simulink model "post_data_run"  (R2020a)
settings: Solver=FixedStepDiscrete  StartTime=0.0  StopTime=P.t_end  FixedStep=P.dt  RelTol=1e-3  EnableMultiTasking=on
PostLoadFcn:
  | load_post_DC
StopFcn:
  | post_post_DC
settings Model: ExtModeTrigDuration=10000  Creator=divad  LastModifiedBy=divad
settings SolverCC: PositivePriorityOrder=on
settings DataIOCC: ReturnWorkspaceOutputs=off
settings OptimizationCC: LifeSpan=inf
settings DebuggingCC: ArithmeticOperatorsInVariantConditions=warning
settings SFSimCC: SimUseLocalCustomCode=off  CustomCodeUndefinedFunction=UseInterfaceOnly
settings RTWCC: Description=QUARC Win64 Target  SystemTargetFile=quarc_win64.tlc  TemplateMakefile=quarc_default_tmf  RTWUseLocalCustomCode=off
settings CodeAppCC: StateflowObjectComments=on
settings STFCustomTargetCC: TargetPreCompLibLocation=C:\PROGRA~3\QUARC\lib\2020a\win64\release  TargetLangStandard=C99 (ISO)  ConcurrentExecutionCompliant=on  GRTInterface=on  SystemTargetFile=quarc_win64.tlc
settings GRTTargetCC: TargetPreCompLibLocation=C:\PROGRA~3\QUARC\lib\2020a\win64\release  ParMdlRefBuildCompliant=off  CompOptLevelCompliant=off  CombineOutputUpdateFcns=off  MatFileLogging=off  CPPClassGenCompliant=off  GRTInterface=on  UseToolchainInfoCompliant=off  ExtMode=on  ExtModeMexFile=quarc_comm
settings ConfigComp: CovMetricSettings=dswe

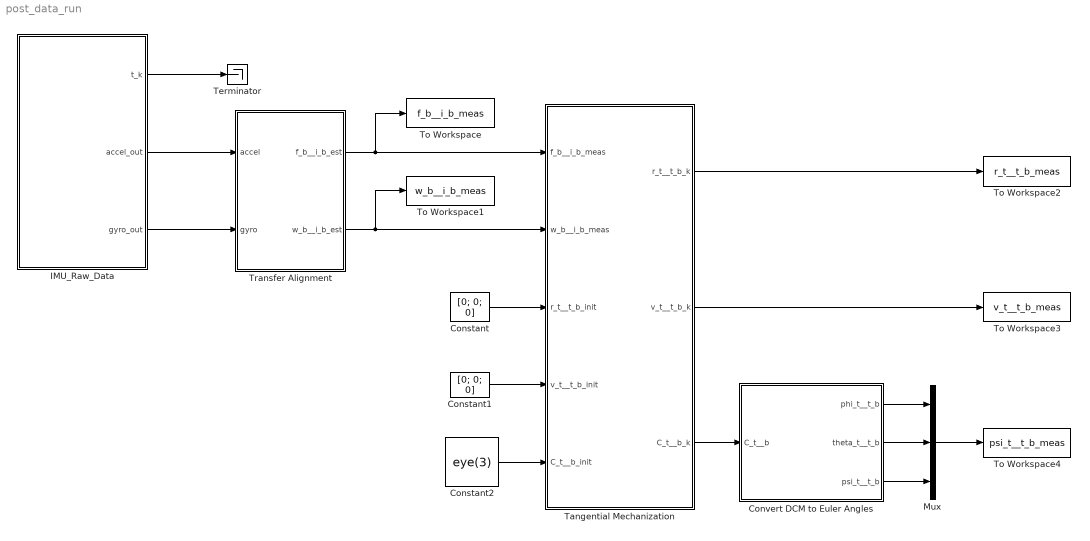
== system post_data_run ==
  Constant : Constant  Value=[0; 0; 0]
  Constant1 : Constant  Value=[0; 0; 0]
  Constant2 : Constant  Value=eye(3)
  Convert DCM to Euler Angles : MATLAB Function  TreatAsAtomicUnit=on
  IMU_Raw_Data : MATLAB Function  TreatAsAtomicUnit=on
  Mux : Mux  Inputs=3
  Tangential Mechanization : Subsystem
  Terminator : Terminator
  To Workspace : ToWorkspace  VariableName=f_b__i_b_meas  SampleTime=-1
      settings: Save2DSignal=2-D array (concatenate along first dimension)
  To Workspace1 : ToWorkspace  VariableName=w_b__i_b_meas  SampleTime=-1
      settings: Save2DSignal=2-D array (concatenate along first dimension)
  To Workspace2 : ToWorkspace  VariableName=r_t__t_b_meas  SampleTime=-1
      settings: Save2DSignal=2-D array (concatenate along first dimension)
  To Workspace3 : ToWorkspace  VariableName=v_t__t_b_meas  SampleTime=-1
      settings: Save2DSignal=2-D array (concatenate along first dimension)
  To Workspace4 : ToWorkspace  VariableName=psi_t__t_b_meas  SampleTime=-1
      settings: Save2DSignal=2-D array (concatenate along first dimension)
  Transfer Alignment : MATLAB Function  TreatAsAtomicUnit=on
  wires:
  IMU_Raw_Data/2(accel_out) -> Transfer Alignment/1(accel)
  IMU_Raw_Data/3(gyro_out) -> Transfer Alignment/2(gyro)
  Transfer Alignment/1(f_b__i_b_est) -> Tangential Mechanization/1(f_b__i_b_meas), To Workspace/1
  Transfer Alignment/2(w_b__i_b_est) -> To Workspace1/1, Tangential Mechanization/2(w_b__i_b_meas)
  IMU_Raw_Data/1(t_k) -> Terminator/1
  Constant/1 -> Tangential Mechanization/3(r_t__t_b_init)
  Constant1/1 -> Tangential Mechanization/4(v_t__t_b_init)
  Constant2/1 -> Tangential Mechanization/5(C_t__b_init)
  Tangential Mechanization/3(C_t__b_k) -> Convert DCM to Euler Angles/1(C_t__b)
  Convert DCM to Euler Angles/1(phi_t__t_b) -> Mux/1
  Convert DCM to Euler Angles/2(theta_t__t_b) -> Mux/2
  Convert DCM to Euler Angles/3(psi_t__t_b) -> Mux/3
  Mux/1 -> To Workspace4/1
  Tangential Mechanization/2(v_t__t_b_k) -> To Workspace3/1
  Tangential Mechanization/1(r_t__t_b_k) -> To Workspace2/1

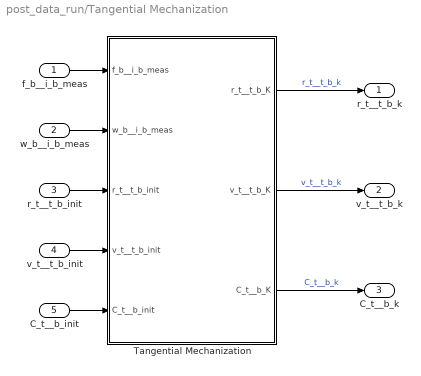
== system post_data_run/Tangential Mechanization ==
  f_b__i_b_meas : Inport
  w_b__i_b_meas : Inport  Port=2
  r_t__t_b_init : Inport  Port=3
  v_t__t_b_init : Inport  Port=4
  C_t__b_init : Inport  Port=5
  Tangential Mechanization : MATLAB Function  TreatAsAtomicUnit=on
  r_t__t_b_k : Outport
  v_t__t_b_k : Outport  Port=2
  C_t__b_k : Outport  Port=3
  wires:
  Tangential Mechanization/3(C_t__b_K) -> C_t__b_k/1  "C_t__b_k"
  f_b__i_b_meas/1 -> Tangential Mechanization/1(f_b__i_b_meas)
  Tangential Mechanization/1(r_t__t_b_K) -> r_t__t_b_k/1  "r_t__t_b_k"
  C_t__b_init/1 -> Tangential Mechanization/5(C_t__b_init)
  v_t__t_b_init/1 -> Tangential Mechanization/4(v_t__t_b_init)
  r_t__t_b_init/1 -> Tangential Mechanization/3(r_t__t_b_init)
  w_b__i_b_meas/1 -> Tangential Mechanization/2(w_b__i_b_meas)
  Tangential Mechanization/2(v_t__t_b_K) -> v_t__t_b_k/1  "v_t__t_b_k"

== matlab function post_data_run/Transfer Alignment ==
  data: accel input; f_b__i_b_est output; gyro input; w_b__i_b_est output; P parameter
function [f_b__i_b_est, w_b__i_b_est] = transfer_alignment(accel, gyro, P)

% Transfer Raw Accel Data into f_b__i_b_meas
accel_est = (eye(3) + P.M_a) \ (accel - P.b_a_FB);
f_b__i_b_est = P.C_b__imu * accel_est;

% Transfer Raw Gyro Data into w_b__i_b_meas
gyro_est = (eye(3) + P.M_g) \ (gyro - P.b_g_FB);
w_b__i_b_est = P.C_b__imu * gyro_est;

== matlab function post_data_run/IMU_Raw_Data ==
  data: t_k output; accel_out output; gyro_out output; P parameter
function [t_k, accel_out, gyro_out] = IMU_Raw_Data(P)

% Initialize k
persistent k

if (isempty(k))
    k = 1;
end

% Return Raw Data Values
t_k = P.t(k);
accel_out = P.accel(k,:)';
gyro_out = P.gyro(k,:)';

% Update Index
k = k + 1;

== matlab function post_data_run/Tangential Mechanization/Tangential Mechanization ==
  data: f_b__i_b_meas input; w_b__i_b_meas input; r_t__t_b_init input; v_t__t_b_init input; C_t__b_init input; r_t__t_b_K output; P parameter; v_t__t_b_K output; C_t__b_K output
function [r_t__t_b_K, v_t__t_b_K, C_t__b_K] = Tan_Mech(f_b__i_b_meas, w_b__i_b_meas, r_t__t_b_init, v_t__t_b_init, C_t__b_init, P)

%% Tan_Mech
% Provides tangential mechanization for kinematic states position, velocity
% and attitude (PVA).  It does this solely based on accel and gyro
% measurements, which come from the IMU block.  The first time step is
% initialized from the ground truth block.  

persistent r_t__t_b_K_1 v_t__t_b_K_1 C_t__b_K_1 g_t__b

% Initialize on First Time Step
if (isempty(r_t__t_b_K_1))
    
    % Use "truth" to initialize on first time step
    r_t__t_b_K = r_t__t_b_init;
    v_t__t_b_K = v_t__t_b_init;
    C_t__b_K   = C_t__b_init;
    
    % Store current values as old values for next iteration
    r_t__t_b_K_1 = r_t__t_b_K;
    v_t__t_b_K_1 = v_t__t_b_K;
    C_t__b_K_1   = C_t__b_K;
    
    % Calculate and store the vector g_t__b
    r_e__e_b = P.r_e__e_t + P.C_e__t*r_t__t_b_init;         % Compute r_e__e_b
    [L_b, lambda_b, h_b] = xyz2llh(r_e__e_b, P);            % Compute the lat, lon, and height
    g_n__b = [0; 0; gravity(L_b, h_b, P)];                  % Compute the acceleration due to gravity
    C_e__n = Lat_Lon_2C_e__n(L_b, lambda_b);                % Compute C_e__n
    g_e__b = C_e__n * g_n__b;                               % Compute the gravity of the body in the {e} frame
    g_t__b = P.C_e__t' * g_e__b;                            % Compute the gravity of the body in the {t} frame 
    
    
    
% Every Other Time Step
else
    
    % C_t__b Rotation Matrix Update 
    if (P.fidelity == 0) % Low Fidelity Method
         
        Ohm_b__i_b_meas = vec2ss(w_b__i_b_meas);
        
        C_t__b_K = C_t__b_K_1*(eye(3) + Ohm_b__i_b_meas*P.dt) - ...
                                              P.Ohm_t__i_e*C_t__b_K_1*P.dt;
                                        
    elseif (P.fidelity == 1) % High Fidelity Method
        
        w_t__t_b = C_t__b_K_1*w_b__i_b_meas - P.C_e__t'*P.w_i__i_e;
        
        % Catch for when w_t__t_b is super super small
        if (norm(w_t__t_b) < 1e-6)
            C_t__b_K = C_t__b_K_1;
        else
            C_t__b_K = double(Rodrigues_k(w_t__t_b * P.dt) * C_t__b_K_1);
        end
        
    end
    
    % f_t__i_b Specific Force Update
    f_t__i_b = C_t__b_K * f_b__i_b_meas;
    
    % a_t__t_b Acceleration Vector Update
    
    a_t__t_b = f_t__i_b + g_t__b - 2*P.Ohm_t__i_e*v_t__t_b_K_1;
    
    % v_t__t_b Velocity Vector Update
    v_t__t_b_K = double(v_t__t_b_K_1 + a_t__t_b*P.dt);
    
    % r_t__t_b Position Vector Update
    r_t__t_b_K = double(r_t__t_b_K_1 + v_t__t_b_K_1*P.dt + a_t__t_b*((P.dt^2)/2));
    
    % Store new PVA as old PVA
    r_t__t_b_K_1 = r_t__t_b_K;
    v_t__t_b_K_1 = v_t__t_b_K;
    C_t__b_K_1   = C_t__b_K;
    
end

== matlab function post_data_run/Convert DCM to Euler Angles ==
  data: C_t__b input; phi_t__t_b output; theta_t__t_b output; psi_t__t_b output
function [phi_t__t_b, theta_t__t_b, psi_t__t_b] = dcm_2_psi(C_t__b)
% Takes in DCM C_t__b and returns ins Euler Angles (phi, theta, psi)
% Function returns angles in order of state estimation requirements

[psi_t__t_b, theta_t__t_b, phi_t__t_b] = dcm2ypr(C_t__b);
